simulink model "ATV_LAB4_SIMU_Q4"  (R2021a)
settings: Solver=VariableStepAuto  StartTime=0.0  StopTime=100  RelTol=1e-3
settings Model: Creator=Home  LastModifiedBy=Home

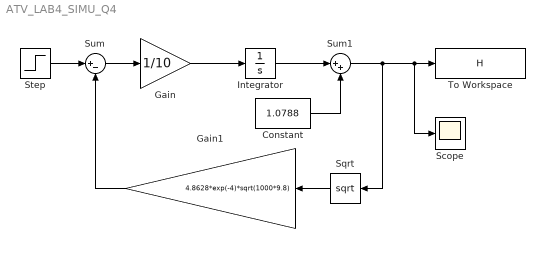
== system ATV_LAB4_SIMU_Q4 ==
  Constant : Constant  Value=1.0788
  Gain : Gain  Gain=1/10
  Gain1 : Gain  Gain=4.8628*exp(-4)*sqrt(1000*9.8)
  Integrator : Integrator
  Scope : Scope
  Sqrt : Sqrt  SaturateOnIntegerOverflow=on
  Step : Step  Time=0.05  Before=0.06  After=0.01  SampleTime=0
  Sum : Sum  Inputs=|+-
  Sum1 : Sum  Inputs=|++
  To Workspace : ToWorkspace  VariableName=H  SampleTime=-1
  wires:
  Sum1/1 -> Scope/1, To Workspace/1, Sqrt/1
  Gain/1 -> Integrator/1
  Integrator/1 -> Sum1/1
  Constant/1 -> Sum1/2
  Step/1 -> Sum/1
  Sum/1 -> Gain/1
  Gain1/1 -> Sum/2
  Sqrt/1 -> Gain1/1
